simulink model "bicyclemodel"  (R2026a)
settings: Solver=VariableStepAuto
settings Model: Creator=eonra  LastModifiedBy=eonra

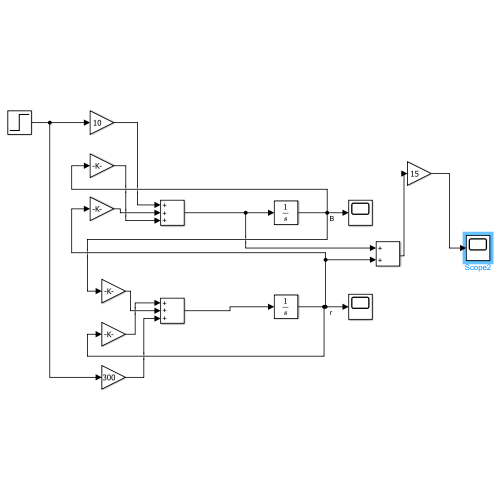
[thumbnail: Simulink's stored preview of the top-level diagram]
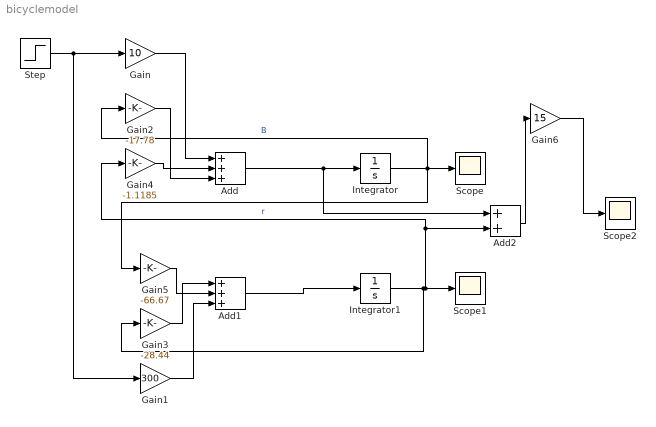
== system bicyclemodel ==
  Add : Sum  Inputs=+++
  Add1 : Sum  Inputs=+++
  Add2 : Sum
  Gain : Gain  Gain=10
  Gain1 : Gain  Gain=300
  Gain2 : Gain  Gain=-17.78
  Gain3 : Gain  Gain=-28.44
  Gain4 : Gain  Gain=-1.1185
  Gain5 : Gain  Gain=-66.67
  Gain6 : Gain  Gain=15
  Integrator : Integrator
  Integrator1 : Integrator
  Scope : Scope
      settings: ActiveDisplayYMinimum=-0.013200928243058109  ActiveDisplayYMaximum=0.015090856433519123
  Scope1 : Scope
      settings: ActiveDisplayYMinimum=-0.11814487855285631  ActiveDisplayYMaximum=1.0633039069757071
  Scope2 : Scope
      settings: ActiveDisplayYMinimum=-1.772679916459839  ActiveDisplayYMaximum=15.954119248138555  DataLoggingVariableName=ScopeData2
  Step : Step  FinalValue=0.0873  SampleTime=0
  wires:
  Integrator/1 -> Gain5/1, Gain2/1, Scope/1  "B"
  Integrator1/1 -> Gain3/1, Add2/2, Gain4/1, Scope1/1  "r"
  Step/1 -> Gain1/1, Gain/1
  Gain1/1 -> Add1/3
  Gain/1 -> Add/1
  Add/1 -> Add2/1, Integrator/1
  Add1/1 -> Integrator1/1
  Gain3/1 -> Add1/1
  Gain2/1 -> Add/3
  Gain5/1 -> Add1/2
  Gain4/1 -> Add/2
  Add2/1 -> Gain6/1
  Gain6/1 -> Scope2/1
